simulink model "faz_bozunumu"  (R2021a)
settings: Solver=FixedStepDiscrete  StartTime=0.0  StopTime=inf  RelTol=1e-3
libraries: simulink x1
settings Model: Creator=Yusuf  LastModifiedBy=Yusuf
settings SolverCC: AlgebraicLoopSolver=TrustRegion  AutoInsertRateTranBlk=on
settings DataIOCC: LimitDataPoints=on  SaveOutput=off  SignalLogging=off  SaveTime=off
settings OptimizationCC: LifeSpan=inf
settings DebuggingCC: AlgebraicLoopMsg=error  SingleTaskRateTransMsg=error  AllowSymbolicDim=off  SFUnexpectedBacktrackingDiag=warning  SFNoUnconditionalDefaultTransitionDiag=warning  SFExecutionAtInitializationDiag=none  SFMachineParentedDataDiag=warning  ArithmeticOperatorsInVariantConditions=warning
settings SFSimCC: SimUseLocalCustomCode=off  CustomCodeUndefinedFunction=UseInterfaceOnly
settings RTWCC: RTWUseLocalCustomCode=off
settings CodeAppCC: StateflowObjectComments=on
settings GRTTargetCC: TargetLangStandard=C89/C90 (ANSI)

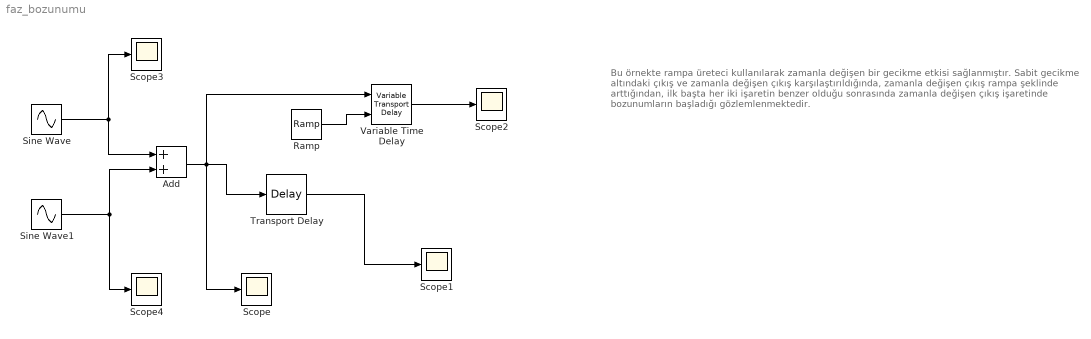
== system faz_bozunumu ==
  note: Bu örnekte rampa üreteci kullanılarak zamanla değişen bir gecikme etkisi sağlanmıştır. Sabit gecikme altındaki çıkış ve zamanla değişen çıkış karşılaştırıldığında, zamanla değişen çıkış rampa şeklinde arttığından, ilk başta her iki işaretin benzer olduğu sonrasında zamanla değişen çıkış işaretinde bozunumların başladığı gözlemlenmektedir.
  Add : Sum
  Ramp : simulink/Sources/Ramp  slope=1  start=0  InitialOutput=0
  Scope{,1..4} (5 alike) : Scope
  Sine Wave : Sin  Amplitude=2  Frequency=5*pi  SampleTime=0.001
  Sine Wave1 : Sin  Frequency=2*pi  SampleTime=0.001
  Transport Delay : TransportDelay
  Variable Time Delay : VariableTransportDelay  MaximumDelay=10
  wires:
  Sine Wave1/1 -> Add/2, Scope4/1
  Sine Wave/1 -> Add/1, Scope3/1
  Add/1 -> Scope/1, Variable Time Delay/1, Transport Delay/1
  Ramp/1 -> Variable Time Delay/2
  Transport Delay/1 -> Scope1/1
  Variable Time Delay/1 -> Scope2/1
